simulink model "ReduceDimStateWatcher"  (R2017b)
settings: Solver=VariableStepAuto  StartTime=0.0  StopTime=40  RelTol=1e-3  EnableMultiTasking=on
settings Model: Creator=B303  LastModifiedBy=zhangxiangrui
settings DataIOCC: LimitDataPoints=on
settings OptimizationCC: LifeSpan=inf
settings DebuggingCC: AllowSymbolicDim=off  SFUnexpectedBacktrackingDiag=warning  SFNoUnconditionalDefaultTransitionDiag=warning  SFExecutionAtInitializationDiag=none
settings ModelReferenceCC: PropagateSignalLabelsOutOfModel=off
settings CodeAppCC: StateflowObjectComments=on
settings GRTTargetCC: TargetLangStandard=C89/C90 (ANSI)
settings ConfigComp: CovMetricSettings=dw  CovHtmlReporting=on  CovSaveCumulativeToWorkspaceVar=on  CovSaveSingleToWorkspaceVar=on  CovExternalEMLEnable=off

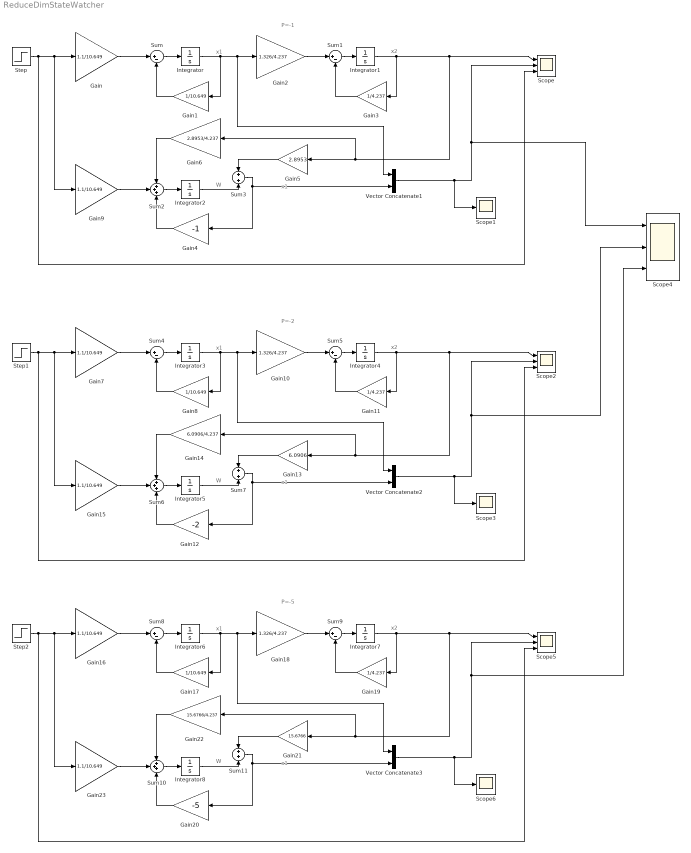
== system ReduceDimStateWatcher ==
  note: x1
  note: x2
  note: W
  note: P=-1
  note: x1
  note: P=-2
  note: x1
  note: x1
  note: W
  note: x2
  note: P=-5
  note: x1
  note: x1
  note: W
  note: x2
  Gain{,7,9,15..16,23} (6 alike) : Gain  Gain=1.1/10.649
  Gain1 : Gain  Gain=1/10.649
  Gain10 : Gain  Gain=1.326/4.237
  Gain11 : Gain  Gain=1/4.237
  Gain12 : Gain  Gain=-2
  Gain13 : Gain  Gain=6.0906
  Gain14 : Gain  Gain=6.0906/4.237
  Gain17 : Gain  Gain=1/10.649
  Gain18 : Gain  Gain=1.326/4.237
  Gain19 : Gain  Gain=1/4.237
  Gain2 : Gain  Gain=1.326/4.237
  Gain20 : Gain  Gain=-5
  Gain21 : Gain  Gain=15.6766
  Gain22 : Gain  Gain=15.6766/4.237
  Gain3 : Gain  Gain=1/4.237
  Gain4 : Gain  Gain=-1
  Gain5 : Gain  Gain=2.8953
  Gain6 : Gain  Gain=2.8953/4.237
  Gain8 : Gain  Gain=1/10.649
  Integrator : Integrator  InitialCondition=2
  Integrator{1..2,4..5,7..8} (6 alike) : Integrator
  Integrator3 : Integrator  InitialCondition=2
  Integrator6 : Integrator  InitialCondition=2
  Scope{,2,4..5} (4 alike) : Scope  NumInputPorts=3
  Scope1 : Scope
  Scope3 : Scope
  Scope6 : Scope
  Step : Step  Time=0  After=3  SampleTime=0
  Step1 : Step  Time=0  After=3  SampleTime=0
  Step2 : Step  Time=0  After=3  SampleTime=0
  Sum{,1,4..5,8..9} (6 alike) : Sum  Inputs=|+-
  Sum10 : Sum  Inputs=+++
  Sum11 : Sum
  Sum2 : Sum  Inputs=+++
  Sum3 : Sum
  Sum6 : Sum  Inputs=+++
  Sum7 : Sum
  Vector Concatenate1 : Concatenate  Mode=Multidimensional array  ConcatenateDimension=2
  Vector Concatenate2 : Concatenate  Mode=Multidimensional array  ConcatenateDimension=2
  Vector Concatenate3 : Concatenate  Mode=Multidimensional array  ConcatenateDimension=2
  wires:
  Sum/1 -> Integrator/1
  Gain/1 -> Sum/1
  Integrator/1 -> Gain1/1, Vector Concatenate1/1, Gain2/1
  Gain1/1 -> Sum/2
  Gain2/1 -> Sum1/1
  Sum1/1 -> Integrator1/1
  Integrator1/1 -> Gain3/1, Gain6/1, Gain5/1, Scope/1
  Gain3/1 -> Sum1/2
  Step/1 -> Scope/3, Gain9/1, Gain/1
  Integrator2/1 -> Sum3/2
  Sum2/1 -> Integrator2/1
  Gain4/1 -> Sum2/3
  Gain9/1 -> Sum2/2
  Gain5/1 -> Sum3/1
  Gain6/1 -> Sum2/1
  Sum3/1 -> Vector Concatenate1/2, Gain4/1
  Vector Concatenate1/1 -> Scope1/1, Scope4/1, Scope/2
  Sum7/1 -> Vector Concatenate2/2, Gain12/1
  Gain7/1 -> Sum4/1
  Gain8/1 -> Sum4/2
  Step1/1 -> Scope2/3, Gain15/1, Gain7/1
  Sum6/1 -> Integrator5/1
  Gain11/1 -> Sum5/2
  Gain13/1 -> Sum7/1
  Gain14/1 -> Sum6/1
  Vector Concatenate2/1 -> Scope3/1, Scope4/2, Scope2/2
  Gain15/1 -> Sum6/2
  Integrator3/1 -> Gain8/1, Vector Concatenate2/1, Gain10/1
  Sum5/1 -> Integrator4/1
  Integrator5/1 -> Sum7/2
  Gain10/1 -> Sum5/1
  Integrator4/1 -> Gain11/1, Gain14/1, Gain13/1, Scope2/1
  Gain12/1 -> Sum6/3
  Sum4/1 -> Integrator3/1
  Sum11/1 -> Vector Concatenate3/2, Gain20/1
  Gain16/1 -> Sum8/1
  Gain17/1 -> Sum8/2
  Step2/1 -> Scope5/3, Gain23/1, Gain16/1
  Sum10/1 -> Integrator8/1
  Gain19/1 -> Sum9/2
  Gain21/1 -> Sum11/1
  Gain22/1 -> Sum10/1
  Vector Concatenate3/1 -> Scope6/1, Scope4/3, Scope5/2
  Gain23/1 -> Sum10/2
  Integrator6/1 -> Gain17/1, Vector Concatenate3/1, Gain18/1
  Sum9/1 -> Integrator7/1
  Integrator8/1 -> Sum11/2
  Gain18/1 -> Sum9/1
  Integrator7/1 -> Gain19/1, Gain22/1, Gain21/1, Scope5/1
  Gain20/1 -> Sum10/3
  Sum8/1 -> Integrator6/1
